simulink subsystem "median7"  (R2021b)
settings: Solver=VariableStepAuto  StartTime=0.0  StopTime=10.0  RelTol=1e-3
settings Model: Creator=dileepan  LastModifiedBy=dileepan

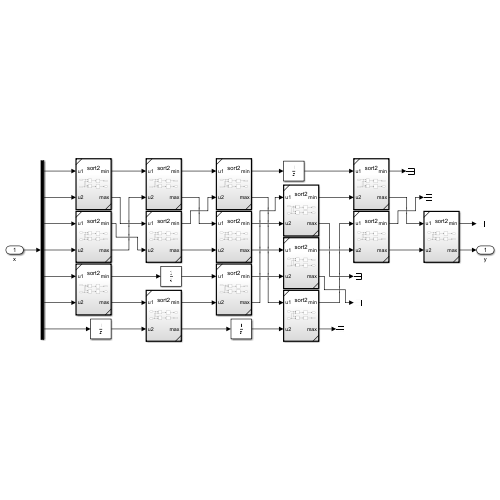
[thumbnail: Simulink's stored preview of the top-level diagram]
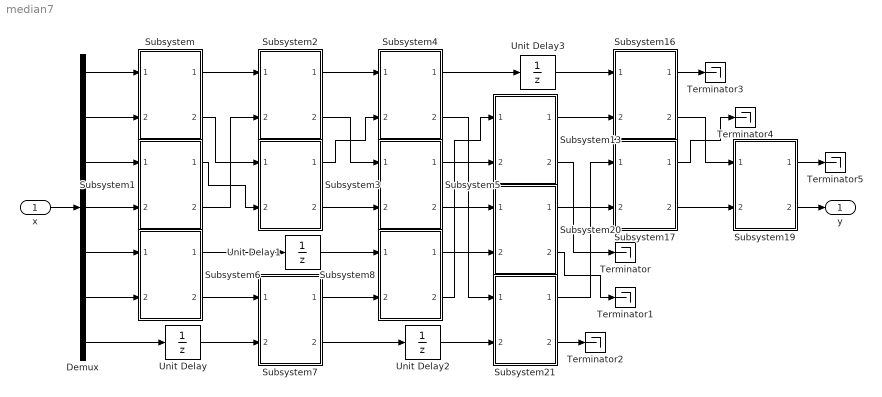
== system median7 ==
  x : Inport
  Demux : Demux  Outputs=7
  Subsystem{,1..8,13,16..17,19..21} (15 alike) : Subsystem  TreatAsAtomicUnit=on  ReferencedSubsystem=sort2
  Terminator{,1..5} (6 alike) : Terminator
  Unit Delay{,1..3} (4 alike) : UnitDelay  SampleTime=-1  HasFrameUpgradeWarning=on
  y : Outport
  wires:
  Subsystem/1 -> Subsystem2/1
  Subsystem1/1 -> Subsystem3/2
  Demux/3 -> Subsystem1/1
  Unit Delay3/1 -> Subsystem16/1
  Unit Delay/1 -> Subsystem7/2
  Subsystem19/2 -> y/1
  Subsystem/2 -> Subsystem3/1
  Demux/2 -> Subsystem/2
  Subsystem16/2 -> Subsystem19/1
  Subsystem21/1 -> Subsystem17/1
  Subsystem4/1 -> Unit Delay3/1
  Subsystem7/2 -> Unit Delay2/1
  Subsystem20/1 -> Subsystem17/2
  Subsystem6/2 -> Subsystem7/1
  Demux/7 -> Unit Delay/1
  Subsystem13/1 -> Subsystem16/2
  Unit Delay1/1 -> Subsystem8/1
  Demux/5 -> Subsystem6/1
  Subsystem7/1 -> Subsystem8/2
  Demux/4 -> Subsystem1/2
  Subsystem6/1 -> Unit Delay1/1
  Subsystem2/2 -> Subsystem5/1
  Subsystem17/2 -> Subsystem19/2
  Subsystem3/1 -> Subsystem4/2
  Demux/6 -> Subsystem6/2
  Subsystem1/2 -> Subsystem2/2
  Subsystem2/1 -> Subsystem4/1
  Subsystem3/2 -> Subsystem5/2
  Demux/1 -> Subsystem/1
  x/1 -> Demux/1
  Subsystem13/2 -> Terminator/1
  Subsystem20/2 -> Terminator1/1
  Subsystem21/2 -> Terminator2/1
  Subsystem16/1 -> Terminator3/1
  Subsystem17/1 -> Terminator4/1
  Subsystem19/1 -> Terminator5/1
  Unit Delay2/1 -> Subsystem21/2
  Subsystem5/2 -> Subsystem20/1
  Subsystem8/1 -> Subsystem20/2
  Subsystem5/1 -> Subsystem13/2
  Subsystem4/2 -> Subsystem21/1
  Subsystem8/2 -> Subsystem13/1
